simulink model "Sobel"  (R2021a)
settings: Solver=VariableStepAuto  StartTime=0.0  StopTime=Ts_480p*2  RelTol=1e-3
InitFcn:
  | Ts = 1e-3;
  | Ts_240p = 402*324*Ts;
  | Ts_480p = 525*800*Ts;
undefined symbols (not defined in the file): gray, Rec, SDTV
libraries: hdlsllib x7, visionhdlio x2, visionhdlconversions x1, dspvision x1
settings Model: Creator=user  LastModifiedBy=user
settings OptimizationCC: BlockReduction=off  ConditionallyExecuteInputs=off  DefaultParameterBehavior=Inlined
settings DebuggingCC: AlgebraicLoopMsg=error
settings HardwareCC: ProdBitPerPointer=32  ProdBitPerSizeT=32  ProdBitPerPtrDiffT=32  ProdLargestAtomicFloat=None  ProdIntDivRoundTo=Undefined  ProdEndianess=Unspecified  ProdWordSize=32  ProdHWDeviceType=ASIC/FPGA->ASIC/FPGA  TargetBitPerPointer=64  TargetBitPerSizeT=64  TargetBitPerPtrDiffT=64  TargetLongLongMode=on  TargetIntDivRoundTo=Zero  TargetEndianess=LittleEndian  TargetWordSize=64  TargetHWDeviceType=Custom Processor->MATLAB Host Computer  ProdEqTarget=off

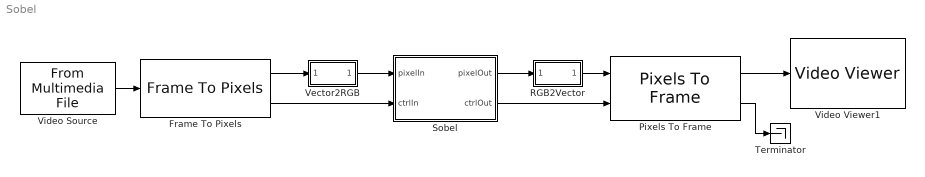
== system Sobel ==
  Frame To Pixels : visionhdlio/Frame To Pixels  NumComponents=3  NumPixels=1  VideoFormat=480p  ActivePixelsPerLine=32  ActiveVideoLines=18  TotalPixelsPerLine=42  TotalVideoLines=28  StartingActiveLine=6  FrontPorch=5  SampleTime=0
      settings: SourceProductBaseCode=VT
  Pixels To Frame : visionhdlio/Pixels To Frame  NumComponents=3  NumPixels=1  VideoFormat=480p  ActivePixelsPerLine=32  ActiveVideoLines=18  TotalPixelsPerLine=42  TotalVideoLines=28
      settings: SourceProductBaseCode=VT
  RGB2Vector : Subsystem
  Sobel : Subsystem  TreatAsAtomicUnit=on
  Terminator : Terminator
  Vector2RGB : Subsystem
  Video Source : dspvision/From Multimedia File  inputFilename=D:\Work\XilFPGAdev\Custom_IP_Cores\SimulinkHDLCoder\testImages\engine_480p.bmp  readRange=[1 Inf]  loop=on  numPlays=inf  outputStreams=Video only  videoDataType=uint8  audioDataType=int16  inheritSampleTime=off  userDefinedSampleTime=Ts_480p  noAudioOutput=off  isIntensityVideo=off  fourcc=RGB  colorVideoFormat=One multidimensional signal  outputEOF=off  dataOrg=Column-major  audioFrameSize=1024  computeAudioFrameSize=off  outSamplingMode=Sample based
  Video Viewer1 : VideoViewer  colormapValue=gray(256)  FigPos=[430.6 726 588 436]
  wires:
  Vector2RGB/1(RGB) -> Sobel/1(pixelIn)
  RGB2Vector/1(RGBVector) -> Pixels To Frame/1
  Frame To Pixels/1 -> Vector2RGB/1(RGBVector)
  Frame To Pixels/2 -> Sobel/2(ctrlIn)
  Pixels To Frame/1 -> Video Viewer1/1
  Pixels To Frame/2 -> Terminator/1
  Video Source/1 -> Frame To Pixels/1
  Sobel/1(pixelOut) -> RGB2Vector/1(RGB)
  Sobel/2(ctrlOut) -> Pixels To Frame/2

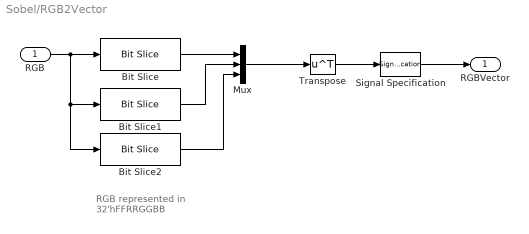
== system Sobel/RGB2Vector ==
  note: RGB represented in
      | 32'hFFRRGGBB
  RGB : Inport
  Bit Slice : hdlsllib/Logic and Bit Operations/Bit Slice  lidx=23  ridx=16
      settings: SourceProductBaseCode=SL
  Bit Slice1 : hdlsllib/Logic and Bit Operations/Bit Slice  lidx=15  ridx=8
      settings: SourceProductBaseCode=SL
  Bit Slice2 : hdlsllib/Logic and Bit Operations/Bit Slice  lidx=7  ridx=0
      settings: SourceProductBaseCode=SL
  Mux : Mux  Inputs=3
  Signal Specification : SignalSpecification
  Transpose : Math  Operator=transpose  SignedPower=on  SaturateOnIntegerOverflow=on
  RGBVector : Outport  VectorParamsAs1DForOutWhenUnconnected=off
  wires:
  Mux/1 -> Transpose/1
  Bit Slice/1 -> Mux/1
  Bit Slice2/1 -> Mux/3
  Bit Slice1/1 -> Mux/2
  RGB/1 -> Bit Slice2/1, Bit Slice1/1, Bit Slice/1
  Transpose/1 -> Signal Specification/1
  Signal Specification/1 -> RGBVector/1

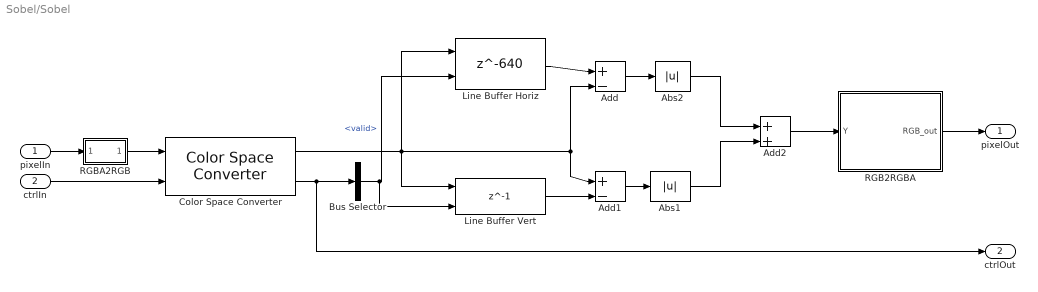
== system Sobel/Sobel ==
  pixelIn : Inport
  ctrlIn : Inport  Port=2
  Abs1 : Abs
  Abs2 : Abs
  Add : Sum  Inputs=+|-  OutDataTypeStr=fixdt(1,12,0)
  Add1 : Sum  Inputs=+|-  OutDataTypeStr=fixdt(1,12,0)
  Add2 : Sum  Inputs=+|+  OutDataTypeStr=fixdt(1,12,0)
  Bus Selector : BusSelector  OutputSignals=valid
  Color Space Converter : visionhdlconversions/Color Space Converter  Conversion=RGB to intensity  ConversionStandard=Rec. 601 (SDTV)  ScanningStandard=1250/50/2:1  SimulateUsing=Code generation
      settings: SourceProductBaseCode=VT
  Line Buffer Horiz : Delay  DelayLength=640  InitialCondition=0  ShowEnablePort=on
      settings: InputPortMap=u0,e6
  Line Buffer Vert : Delay  DelayLength=1  InitialCondition=0  ShowEnablePort=on
      settings: InputPortMap=u0,e6
  RGB2RGBA : MATLAB Function  TreatAsAtomicUnit=on
  RGBA2RGB : Subsystem
  pixelOut : Outport
  ctrlOut : Outport  Port=2  VectorParamsAs1DForOutWhenUnconnected=off
  wires:
  ctrlIn/1 -> Color Space Converter/2
  pixelIn/1 -> RGBA2RGB/1(RGBA)
  Color Space Converter/2 -> Bus Selector/1, ctrlOut/1
  RGBA2RGB/1(RGB) -> Color Space Converter/1
  Abs2/1 -> Add2/1
  RGB2RGBA/1(RGB_out) -> pixelOut/1
  Add1/1 -> Abs1/1
  Add/1 -> Abs2/1
  Color Space Converter/1 -> Line Buffer Horiz/1, Add/2, Add1/1, Line Buffer Vert/1
  Line Buffer Vert/1 -> Add1/2
  Abs1/1 -> Add2/2
  Add2/1 -> RGB2RGBA/1(Y)
  Bus Selector/1 -> Line Buffer Vert/2, Line Buffer Horiz/2  "<valid>"
  Line Buffer Horiz/1 -> Add/1

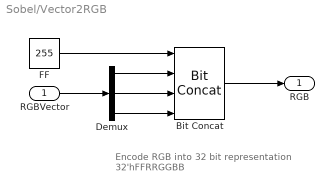
== system Sobel/Vector2RGB ==
  note: Encode RGB into 32 bit representation
      | 32'hFFRRGGBB
  RGBVector : Inport
  Bit Concat : hdlsllib/Logic and Bit Operations/Bit Concat  numInputs=4
  Demux : Demux  Outputs=3
  FF : Constant  Value=255  OutDataTypeStr=uint8  SampleTime=Ts
  RGB : Outport  VectorParamsAs1DForOutWhenUnconnected=off
  wires:
  Bit Concat/1 -> RGB/1
  RGBVector/1 -> Demux/1
  FF/1 -> Bit Concat/1
  Demux/1 -> Bit Concat/2
  Demux/2 -> Bit Concat/3
  Demux/3 -> Bit Concat/4

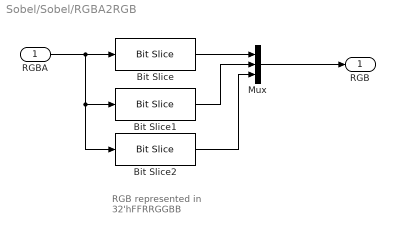
== system Sobel/Sobel/RGBA2RGB ==
  note: RGB represented in
      | 32'hFFRRGGBB
  RGBA : Inport
  Bit Slice : hdlsllib/Logic and Bit Operations/Bit Slice  lidx=23  ridx=16
      settings: SourceProductBaseCode=SL
  Bit Slice1 : hdlsllib/Logic and Bit Operations/Bit Slice  lidx=15  ridx=8
      settings: SourceProductBaseCode=SL
  Bit Slice2 : hdlsllib/Logic and Bit Operations/Bit Slice  lidx=7  ridx=0
      settings: SourceProductBaseCode=SL
  Mux : Mux  Inputs=3
  RGB : Outport  VectorParamsAs1DForOutWhenUnconnected=off
  wires:
  Bit Slice/1 -> Mux/1
  Bit Slice2/1 -> Mux/3
  Bit Slice1/1 -> Mux/2
  RGBA/1 -> Bit Slice2/1, Bit Slice1/1, Bit Slice/1
  Mux/1 -> RGB/1

== matlab function Sobel/RGB2RGBA ==
  data: Y input; RGB_out output
function RGB_out = Concat_Sig(Y)
% 32'hAARRBBGG
Y = Y *2;
Rd = fi(Y, 0, 8, 0);
Gr = fi(Y, 0, 8, 0);
Bl = fi(Y, 0, 8, 0);
AA = fi(255, 0, 8, 0);
RGB_out = bitconcat(AA,Rd,Gr,Bl);
